simulink model "AllPass_ParaEQ"  (R2018b)
settings: Solver=FixedStepAuto  StartTime=0.0  StopTime=inf  RelTol=1e-3  EnableMultiTasking=on
libraries: stm32f769ilib x2
settings Model: SimulationMode=external  Creator=Pemmavit  LastModifiedBy=hpong
settings OptimizationCC: EnhancedBackFolding=on  PassReuseOutputArgsAs=Individual arguments  MaxStackSize=64  OptimizeBlockOrder=speed  DifferentSizesBufferReuse=on  OptimizationCustomize=off
settings DebuggingCC: ParameterTunabilityLossMsg=error
settings HardwareCC: ProdBitPerPointer=32  ProdBitPerSizeT=32  ProdBitPerPtrDiffT=32  ProdLargestAtomicInteger=Long  ProdLargestAtomicFloat=Double  ProdWordSize=32  ProdHWDeviceType=ARM Compatible->ARM Cortex
settings SFSimCC: MATLABDynamicMemAlloc=off
settings RTWCC: SystemTargetFile=ert.tlc  HardwareBoard=STM32F769I-Discovery  TemplateMakefile=ert_default_tmf  GenerateReport=on  Toolchain=GNU Tools for ARM Embedded Processors  IncludeHyperlinkInReport=on  LaunchReport=on  GenerateTraceInfo=on  GenerateTraceReport=on  GenerateTraceReportSl=on  GenerateTraceReportSf=on  GenerateTraceReportEml=on
settings CodeAppCC: ForceParamTrailComments=on  IgnoreCustomStorageClasses=off  OperatorAnnotations=on  SimulinkDataObjDesc=on  SFDataObjDesc=on  InsertBlockDesc=on
settings ERTTargetCC: CodeReplacementLibrary=ARM Cortex-M (CMSIS)

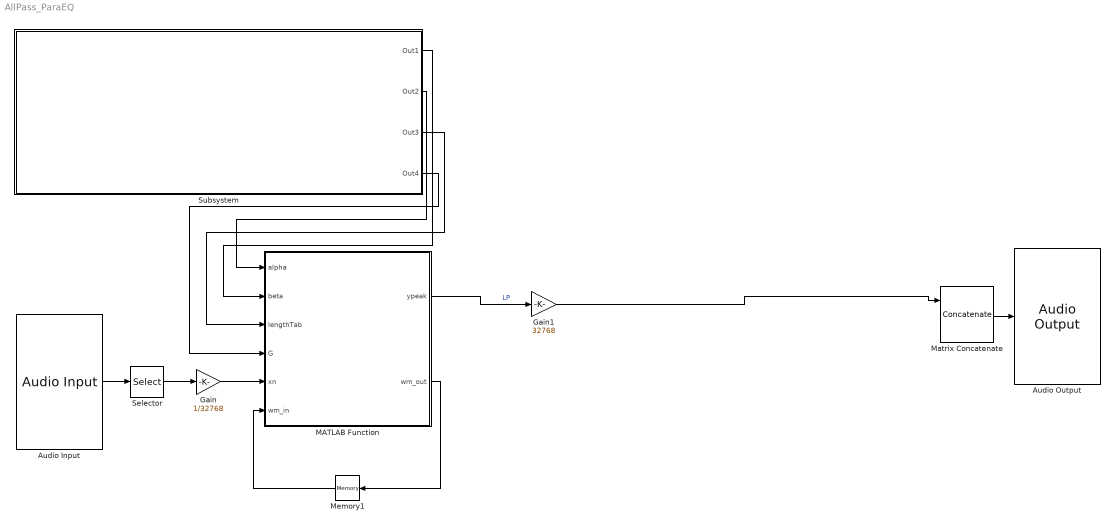
== system AllPass_ParaEQ ==
  Audio Input : stm32f769ilib/Audio Input  InputDevice=LineIn  SamplingFreq=44100  NumCh=2  FrameSize=4096
      settings: SourceProductName=Embedded Coder Support Package for STMicroelectronics Discovery Boards  SourceProductBaseCode=STMICRODIS
  Audio Output : stm32f769ilib/Audio Output  OutputDevice=Headphone  SamplingFreq=44100  Volume=64
      settings: SourceProductName=Embedded Coder Support Package for STMicroelectronics Discovery Boards  SourceProductBaseCode=STMICRODIS
  Gain : Gain  Gain=1/32768  ParamDataTypeStr=double  OutDataTypeStr=double
  Gain1 : Gain  Gain=32768  ParamDataTypeStr=int16  OutDataTypeStr=int16
  MATLAB Function : MATLAB Function  TreatAsAtomicUnit=on
  Matrix Concatenate : Concatenate  Mode=Multidimensional array  ConcatenateDimension=2
  Memory1 : Memory  InitialCondition=[0 0;0 0;0 0;0 0;0 0]  InheritSampleTime=on
  Selector : Selector  NumberOfDimensions=2  InputPortWidth=3  IndexOptions=Select all,Index vector (dialog)  Indices=[1 3],1  OutputSizes=1,1
  Subsystem : Subsystem
  wires:
  Audio Input/1 -> Selector/1
  Selector/1 -> Gain/1
  Matrix Concatenate/1 -> Audio Output/1
  Gain/1 -> MATLAB Function/5(xn)
  MATLAB Function/2(wm_out) -> Memory1/1
  Memory1/1 -> MATLAB Function/6(wm_in)
  MATLAB Function/1(ypeak) -> Gain1/1  "LP"
  Gain1/1 -> Matrix Concatenate/1
  Subsystem/1(Out1) -> MATLAB Function/2(beta)
  Subsystem/2(Out2) -> MATLAB Function/1(alpha)
  Subsystem/3(Out3) -> MATLAB Function/3(lengthTab)
  Subsystem/4(Out4) -> MATLAB Function/4(G)

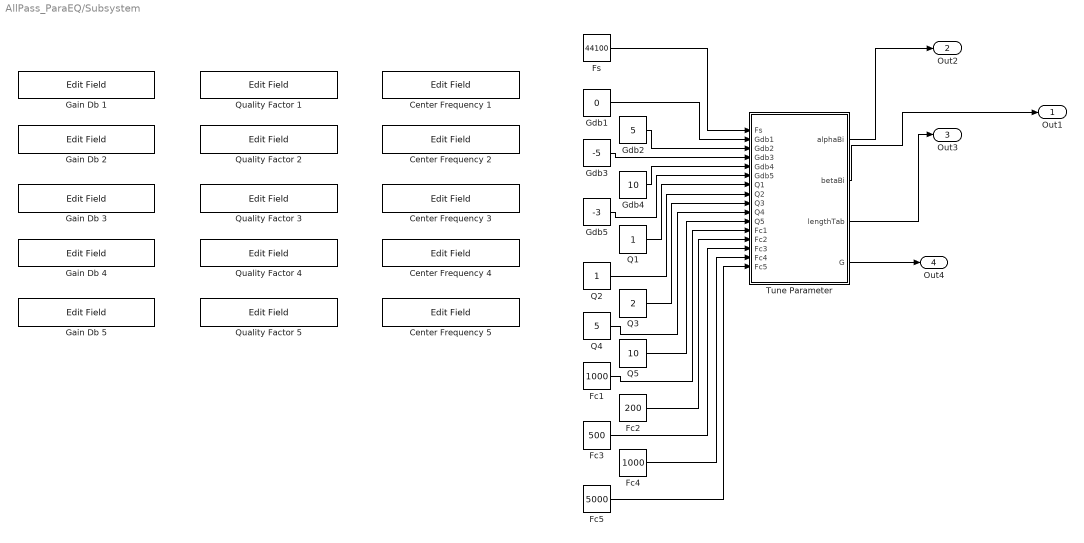
== system AllPass_ParaEQ/Subsystem ==
  Center Frequency 1 : EditField  WebBlockId=93  LabelPosition=Hide  ShowInitialText=on  Alignment=Center
  Center Frequency 2 : EditField  WebBlockId=94  LabelPosition=Hide  ShowInitialText=on  Alignment=Center
  Center Frequency 3 : EditField  WebBlockId=95  LabelPosition=Hide  ShowInitialText=on  Alignment=Center
  Center Frequency 4 : EditField  WebBlockId=96  LabelPosition=Hide  ShowInitialText=on  Alignment=Center
  Center Frequency 5 : EditField  WebBlockId=97  LabelPosition=Hide  ShowInitialText=on  Alignment=Center
  Fc1 : Constant  Value=1000
  Fc2 : Constant  Value=200
  Fc3 : Constant  Value=500
  Fc4 : Constant  Value=1000
  Fc5 : Constant  Value=5000
  Fs : Constant  Value=44100
  Gain Db 1 : EditField  WebBlockId=80  LabelPosition=Hide  ShowInitialText=on  Alignment=Center
  Gain Db 2 : EditField  WebBlockId=81  LabelPosition=Hide  ShowInitialText=on  Alignment=Center
  Gain Db 3 : EditField  WebBlockId=84  LabelPosition=Hide  ShowInitialText=on  Alignment=Center
  Gain Db 4 : EditField  WebBlockId=85  LabelPosition=Hide  ShowInitialText=on  Alignment=Center
  Gain Db 5 : EditField  WebBlockId=86  LabelPosition=Hide  ShowInitialText=on  Alignment=Center
  Gdb1 : Constant  Value=0
  Gdb2 : Constant  Value=5
  Gdb3 : Constant  Value=-5
  Gdb4 : Constant  Value=10
  Gdb5 : Constant  Value=-3
  Q1 : Constant
  Q2 : Constant
  Q3 : Constant  Value=2
  Q4 : Constant  Value=5
  Q5 : Constant  Value=10
  Quality Factor 1 : EditField  WebBlockId=87  LabelPosition=Hide  ShowInitialText=on  Alignment=Center
  Quality Factor 2 : EditField  WebBlockId=88  LabelPosition=Hide  ShowInitialText=on  Alignment=Center
  Quality Factor 3 : EditField  WebBlockId=90  LabelPosition=Hide  ShowInitialText=on  Alignment=Center
  Quality Factor 4 : EditField  WebBlockId=91  LabelPosition=Hide  ShowInitialText=on  Alignment=Center
  Quality Factor 5 : EditField  WebBlockId=92  LabelPosition=Hide  ShowInitialText=on  Alignment=Center
  Tune Parameter : MATLAB Function  TreatAsAtomicUnit=on
  Out1 : Outport
  Out2 : Outport  Port=2
  Out3 : Outport  Port=3
  Out4 : Outport  Port=4
  wires:
  Gdb1/1 -> Tune Parameter/2(Gdb1)
  Gdb2/1 -> Tune Parameter/3(Gdb2)
  Gdb3/1 -> Tune Parameter/4(Gdb3)
  Gdb4/1 -> Tune Parameter/5(Gdb4)
  Gdb5/1 -> Tune Parameter/6(Gdb5)
  Q1/1 -> Tune Parameter/7(Q1)
  Q2/1 -> Tune Parameter/8(Q2)
  Q3/1 -> Tune Parameter/9(Q3)
  Tune Parameter/2(betaBi) -> Out1/1
  Fs/1 -> Tune Parameter/1(Fs)
  Q4/1 -> Tune Parameter/10(Q4)
  Q5/1 -> Tune Parameter/11(Q5)
  Fc1/1 -> Tune Parameter/12(Fc1)
  Fc2/1 -> Tune Parameter/13(Fc2)
  Fc3/1 -> Tune Parameter/14(Fc3)
  Fc4/1 -> Tune Parameter/15(Fc4)
  Fc5/1 -> Tune Parameter/16(Fc5)
  Tune Parameter/1(alphaBi) -> Out2/1
  Tune Parameter/3(lengthTab) -> Out3/1
  Tune Parameter/4(G) -> Out4/1

== matlab function AllPass_ParaEQ/Subsystem/Tune Parameter ==
  data: alphaBi output; Fs input; Gdb1 input; betaBi output; Gdb2 input; Gdb3 input; Gdb4 input; Gdb5 input; Q1 input; Q2 input; Q3 input; Q4 input; Q5 input; Fc1 input; Fc2 input; Fc3 input; Fc4 input; Fc5 input; lengthTab output; G output
function [alphaBi,betaBi,lengthTab,G] = fcn(Fs,Gdb1,Gdb2,Gdb3,Gdb4,Gdb5,Q1,Q2,Q3,Q4,Q5,Fc1,Fc2,Fc3,Fc4,Fc5)
f0 = [Fc1 Fc2 Fc3 Fc4 Fc5];
G_dB = [Gdb1 Gdb2 Gdb3 Gdb4 Gdb5];
Q = [Q1 Q2 Q3 Q4 Q5];

G = 10.^(G_dB./20);
wc = 2*pi.*f0./Fs;
Bw = wc./Q;
% fl = logspace(0,log10(Fs/2),1000);

lengthTab = length(f0);
betaBi = cos(wc);
alphaBi = (sqrt(G)-tan(Bw./2))./(sqrt(G)+tan(Bw./2));
% 
% d1 = -(1+alphaBi).*betaBi;
% d2 = alphaBi;
% Glp = 0.25.*(1-betaBi).*(1+alphaBi);
% Ghp = 0.25.*(1+betaBi).*(1+alphaBi);
% Gbp = 0.5.*(1-alphaBi);
% 
% a = [ones(1,length(f0)) ; d1 ; d2];
% 
% H_Bi = zeros(1000,length(f0))+ ones(1000,length(f0))*1j;
% bbp = zeros(3,length(f0));
% blp = zeros(3,length(f0));
% bhp = zeros(3,length(f0));
% for i=1:length(f0)
%     bbp(:,i) = [1 ; 0 ; -1].*Gbp(i);
%     blp(:,i) = [1 ; 2 ; 1].*Glp(i);
%     bhp(:,i) = [1 ; -2 ; 1].*Ghp(i);
%     [H_Bi(:,i),fl] = freqz(bhp(:,i)+blp(:,i)+bbp(:,i)*G(i) ,a(:,i),1000,44100);
% end
% Freq_Resp = H_Bi(:,1).* H_Bi(:,2).* H_Bi(:,3).* H_Bi(:,4).* H_Bi(:,5);
% 
% semilogx(fl,20*log10(abs(Freq_Resp)));
% xlim([20 Fs/2]);
% grid on

== matlab function AllPass_ParaEQ/MATLAB Function ==
  data: alpha input; beta input; lengthTab input; G input; ypeak output; xn input; wm_in input; wm_out output
function [ypeak, wm_out] = iir_test(alpha,beta,lengthTab,G, xn,wm_in)
sample_per_frame = 4096;

d1 = -(1+alpha).*beta;
d2 = alpha;
Glp = 0.25.*(1-beta).*(1+alpha);
Ghp = 0.25.*(1+beta).*(1+alpha);
Gbp = 0.5.*(1-alpha);


wn = [zeros(5,1) wm_in];
ytemp = zeros(1,sample_per_frame);
ypeak = zeros(1,sample_per_frame);
i=1;
% for i = 1:lengthTab
    for n = 1:sample_per_frame
        
        wn(i,1) = xn(n) - wn(i,2)*d1(i) - wn(i,3)*d2(i);
       
        ylp = (wn(i,1) + wn(i,3) + 2*wn(i,2))*Glp(i);
        yhp = (wn(i,1) + wn(i,3) - 2*wn(i,2))*Ghp(i);
        ybp = (wn(i,1) - wn(i,3))*Gbp(i)*G(i);
%         ypeak(n) = ylp + yhp + ybp;
ypeak(n) = xn(n)/2;
%         xn(n) = ytemp(n);
%         if i == lengthTab
%             ypeak(n) = ytemp(n);
%         end
    end
    wn(i,3) = wn(i,2);
    wn(i,2) = wn(i,1);
% end
wm_out = wn(:,1:2);
%-------------------------------------------
